simulink model "rotationalkinematicseuler"  (R2023a)
settings: Solver=VariableStepAuto  StartTime=0.0  StopTime=10.0  RelTol=1e-3
undefined symbols (not defined in the file): pitch, roll, yaw
settings Model: Creator=prafulsigdel  LastModifiedBy=prafulsigdel

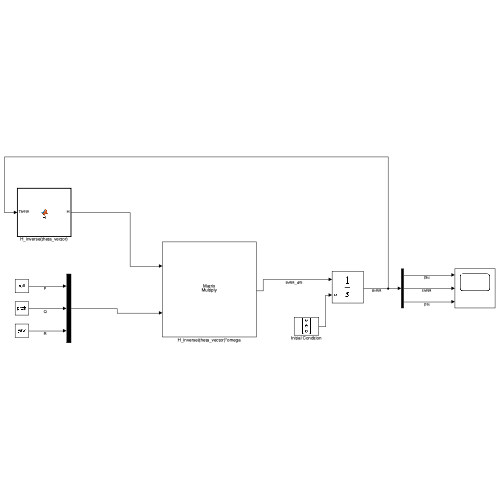
[thumbnail: Simulink's stored preview of the top-level diagram]
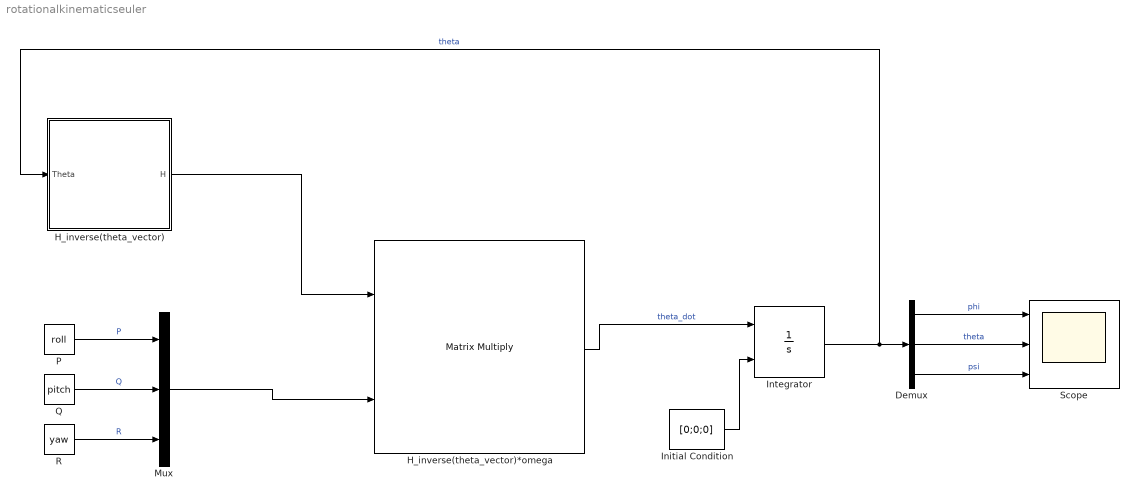
== system rotationalkinematicseuler ==
  Demux : Demux  Outputs=3
  H_inverse(theta_vector) : MATLAB Function  TreatAsAtomicUnit=on
  H_inverse(theta_vector)*omega : Product  Multiplication=Matrix(*)
  Initial Condition : Constant  Value=[0;0;0]  VectorParams1D=off
  Integrator : Integrator  InitialConditionSource=external
  Mux : Mux  Inputs=3
  P : Constant  Value=roll
  Q : Constant  Value=pitch
  R : Constant  Value=yaw
  Scope : Scope  NumInputPorts=3
  wires:
  H_inverse(theta_vector)/1(H) -> H_inverse(theta_vector)*omega/1
  H_inverse(theta_vector)*omega/1 -> Integrator/1  "theta_dot"
  Initial Condition/1 -> Integrator/2
  Integrator/1 -> H_inverse(theta_vector)/1(Theta), Demux/1  "theta"
  P/1 -> Mux/1  "P"
  Q/1 -> Mux/2  "Q"
  Mux/1 -> H_inverse(theta_vector)*omega/2
  R/1 -> Mux/3  "R"
  Demux/1 -> Scope/1  "phi"
  Demux/2 -> Scope/2  "theta"
  Demux/3 -> Scope/3  "psi"

== matlab function rotationalkinematicseuler/H_inverse(theta_vector) ==
  data: Theta input; H output
function H = H(Theta)

% Create a H_inverse 3*3 matrix by unpacking theta
phi = Theta(1);
theta = Theta(2);
psi = Theta(3);

H = [1 tan(theta)*sin(phi) tan(theta)*cos(phi);
    0 cos(phi) -sin(phi);
    0 sin(phi)/cos(theta) cos(phi)/cos(theta)];
